simulink model "TestingHILSimulation"  (R2024b)
settings: Solver=FixedStepAuto  StartTime=0.0  StopTime=inf  FixedStep=0.05  RelTol=1e-3
model workspace (MAT data in the model file):
  NumRxValues = 3
  NumTxVariables = 3
undefined symbols (not defined in the file or in its folder): f
libraries: instrumentlib x2
settings Model: Creator=natha  LastModifiedBy=natha

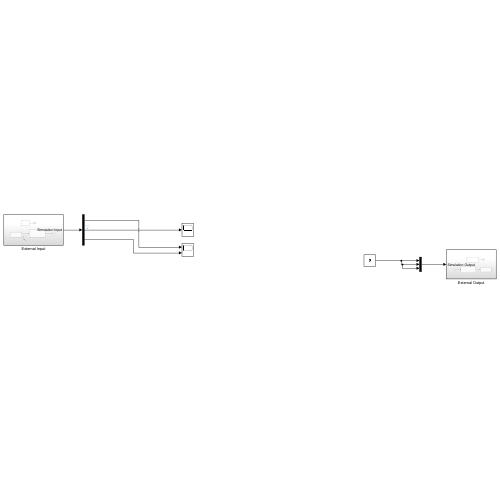
[thumbnail: Simulink's stored preview of the top-level diagram]
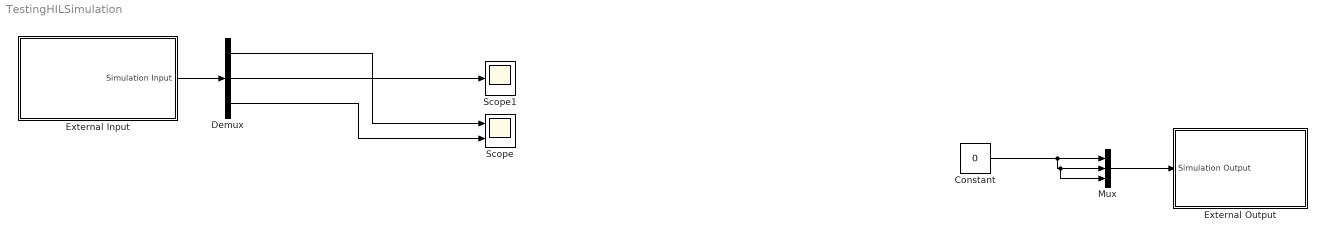
== system TestingHILSimulation ==
  Constant : Constant  Value=0
  Demux : Demux  Outputs=NumRxValues
  External Input : Subsystem
  External Output : Subsystem
  Mux : Mux  Inputs=NumTxVariables
  Scope : Scope  NumInputPorts=2
  Scope1 : Scope
  wires:
  External Input/1(Simulation Input) -> Demux/1
  Mux/1 -> External Output/1(Simulation Output)
  Constant/1 -> Mux/3, Mux/2, Mux/1
  Demux/1 -> Scope/1
  Demux/3 -> Scope/2
  Demux/2 -> Scope1/1

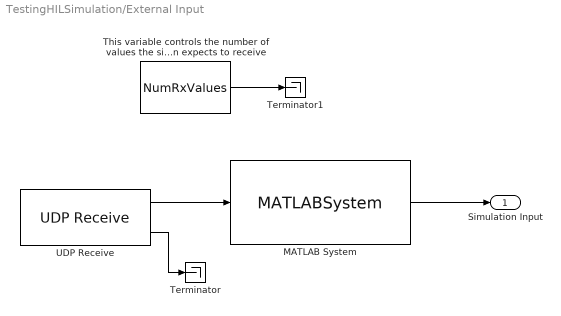
== system TestingHILSimulation/External Input ==
  MATLAB System : MATLABSystem  System=BytesToFloats  NumValues=NumRxValues  SimulateUsing=Code generation
      mask Type: BytesToFloats
      mask Display:
      | disp('BytesToFloats');
      | port_label('input',1,'bytes');
      | port_label('output',1,'floatValues');
  Terminator : Terminator
  Terminator1 : Terminator
  This variable controls the number of values the simulation expects to receive : Constant  Value=NumRxValues
  UDP Receive : instrumentlib/UDP Receive  LocalAddress=127.0.0.1  LocalPort=25000  EnablePortSharing=off  Host=localhost  Port=25001  GetLatestData=on  DataSize=[ 1, 8*NumRxValues ]  DataType=uint8  ASCIIFormatting=%f,  Terminator=LF  CustomTerminator=10  ByteOrder=big-endian  EnableBlockingMode=off  Timeout=10  SampleTime=0.05  SimulateUsing=Interpreted execution
  Simulation Input : Outport
  wires:
  UDP Receive/1 -> MATLAB System/1
  MATLAB System/1 -> Simulation Input/1
  UDP Receive/2 -> Terminator/1
  This variable controls the number of values the simulation expects to receive/1 -> Terminator1/1

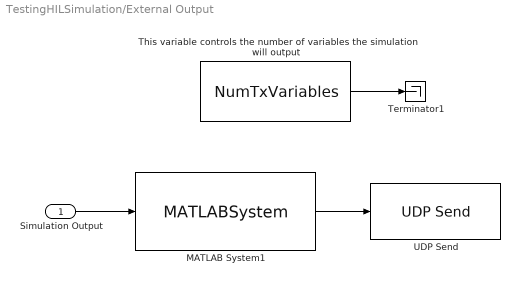
== system TestingHILSimulation/External Output ==
  Simulation Output : Inport
  MATLAB System1 : MATLABSystem  System=FloatsToBytes  NumValues=NumTxVariables  SimulateUsing=Code generation
      mask Type: FloatsToBytes
      mask Display:
      | disp('FloatsToBytes');
      | port_label('input',1,'floatValues');
      | port_label('output',1,'bytes');
  Terminator1 : Terminator
  This variable controls the number of variables the simulation will output : Constant  Value=NumTxVariables
  UDP Send : instrumentlib/UDP Send  Host=127.0.0.1  Port=25001  LocalAddress=127.0.0.1  LocalPort=25000  EnablePortSharing=off  OutputDatagramPacketSize=8 * NumTxVariables  ByteOrder=big-endian  EnableBlockingMode=off  SimulateUsing=Interpreted execution
  wires:
  MATLAB System1/1 -> UDP Send/1
  Simulation Output/1 -> MATLAB System1/1
  This variable controls the number of variables the simulation will output/1 -> Terminator1/1
